simulink model "EPSsim"  (R2020b)
settings: Solver=VariableStepAuto  StartTime=0.0  StopTime=10.0  RelTol=1e-3
settings Model: Creator=Chronos  LastModifiedBy=Chronos

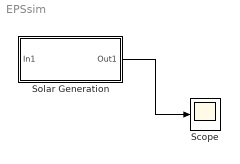
== system EPSsim ==
  Scope : Scope
  Solar Generation : Subsystem
  wires:
  Solar Generation/1(Out1) -> Scope/1

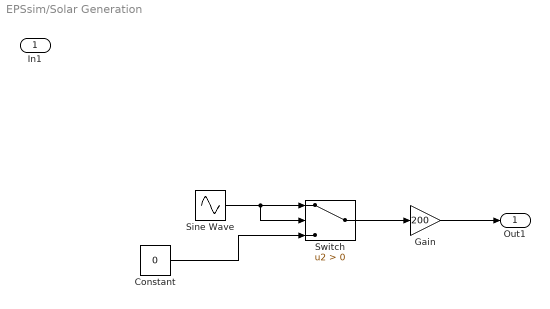
== system EPSsim/Solar Generation ==
  In1 : Inport
  Constant : Constant  Value=0
  Gain : Gain  Gain=200
  Sine Wave : Sin  SampleTime=0
  Switch : Switch  Criteria=u2 > Threshold
  Out1 : Outport
  wires:
  Constant/1 -> Switch/3
  Sine Wave/1 -> Switch/1, Switch/2
  Switch/1 -> Gain/1
  Gain/1 -> Out1/1
